simulink model "e02_MtrCtrl_Pst"  (R2024a)
settings: Solver=FixedStepDiscrete  StartTime=0.0  StopTime=1  FixedStep=mSim.dTime  MaxStep=Define.sModelSampleTime  RelTol=7.1420e-05
undefined symbols (not defined in the file): CnstCnst, E02ITDC, E02PST
libraries: simulink x6, Lib_LPF x3
settings Model: Creator=user  LastModifiedBy=admin
settings SolverCC: MaxConsecutiveZCs=10000  ZeroCrossAlgorithm=Adaptive  AlgebraicLoopSolver=TrustRegion
settings DataIOCC: SaveOutput=off  DSMLogging=off  InspectSignalLogs=on  SaveTime=off  SignalLoggingName=logsout_Validator
settings OptimizationCC: BlockReduction=off  DefaultParameterBehavior=Inlined  UseDivisionForNetSlopeComputation=UseDivisionForReciprocalsOfIntegersOnly  GainParamInheritBuiltInType=on  UseFloatMulNetSlope=on  DefaultUnderspecifiedDataType=single  InlineInvariantSignals=on  BitwiseOrLogicalOp=Logical operator  PassReuseOutputArgsAs=Individual arguments  EfficientFloat2IntCast=on  LifeSpan=Inf  OptimizeBlockOrder=speed  DifferentSizesBufferReuse=on  EfficientTunableParamExpr=on
settings DebuggingCC: SignalInfNanChecking=error  SignalRangeChecking=error  ReadBeforeWriteMsg=EnableAllAsError  WriteAfterWriteMsg=EnableAllAsError  WriteAfterReadMsg=EnableAllAsError  AlgebraicLoopMsg=error  ArtificialAlgebraicLoopMsg=error  SaveWithDisabledLinksMsg=error  SaveWithParameterizedLinksMsg=error  BlockPriorityViolationMsg=error  SolverPrmCheckMsg=error  InheritedTsInSrcMsg=error  SingleTaskRateTransMsg=error  TasksWithSamePriorityMsg=error  SigSpecEnsureSampleTimeMsg=error  CheckMatrixSingularityMsg=error  IntegerOverflowMsg=error  ParameterUnderflowMsg=error  ParameterPrecisionLossMsg=error  ParameterTunabilityLossMsg=error  UnderSpecifiedDataTypeMsg=error  UnnecessaryDatatypeConvMsg=warning  VectorMatrixConversionMsg=error  SignalLabelMismatchMsg=error  UnconnectedInputMsg=error  UnconnectedOutputMsg=error  UnconnectedLineMsg=error  SFcnCompatibilityMsg=error  UniqueDataStoreMsg=error  BusObjectLabelMismatch=error  RootOutportRequireBusObject=error  AssertControl=DisableAll  ModelReferenceIOMismatchMessage=error  UnknownTsInhSupMsg=error  ModelReferenceDataLoggingMessage=error  ModelReferenceSymbolNameMessage=none  StateNameClashWarn=warning  StrictBusMsg=ErrorOnBusTreatedAsVector  NonBusSignalsTreatedAsBus=error  SFInvalidInputDataAccessInChartInitDiag=error  SFTransitionOutsideNaturalParentDiag=error  SFUnreachableExecutionPathDiag=error  SFUndirectedBroadcastEventsDiag=error  SFTransitionActionBeforeConditionDiag=error  SFTemporalDelaySmallerThanSampleTimeDiag=error  SFSelfTransitionDiag=error  SFExecutionAtInitializationDiag=error  IntegerSaturationMsg=error  UnitsInconsistencyMsg=none  VariantConditionMismatch=error
settings HardwareCC: ProdBitPerChar=16  ProdBitPerInt=16  ProdBitPerPointer=32  ProdBitPerSizeT=32  ProdBitPerPtrDiffT=32  ProdLargestAtomicInteger=Integer  ProdLargestAtomicFloat=None  ProdWordSize=16  ProdLongLongMode=on  ProdHWDeviceType=Texas Instruments->C2000
settings ModelReferenceCC: EnableRefExpFcnMdlSchedulingChecks=on  ModelReferenceNumInstancesAllowed=Single
settings SFSimCC: SimUseLocalCustomCode=off  CompileTimeRecursionLimit=0  EnableRuntimeRecursion=off  MATLABDynamicMemAlloc=off  CustomCodeUndefinedFunction=UseInterfaceOnly
settings RTWCC: Description=Embedded Coder  SystemTargetFile=ert.tlc  GenCodeOnly=on  TemplateMakefile=ert_default_tmf  GenerateReport=on  RTWUseLocalCustomCode=off  BuildConfiguration=Faster Runs  IncludeHyperlinkInReport=on  LaunchReport=on  GenerateTraceInfo=on  GenerateTraceReport=on  GenerateTraceReportSl=on  GenerateTraceReportSf=on  GenerateWebview=on  GenerateCodeMetricsReport=on  GenerateCodeReplacementReport=on  GPUComputeCapability=3.5  DLArmComputeVersion=19.05
settings CodeAppCC: ForceParamTrailComments=on  IgnoreCustomStorageClasses=off  MATLABFcnDesc=on  MangleLength=4  CustomSymbolStrGlobalVar=GvE02$N$M  CustomSymbolStrType=StrE02$N$M  CustomSymbolStrFcn=$N$M$F  CustomSymbolStrMacro=$N$M  DefineNamingRule=UpperCase  ParamNamingRule=UpperCase  SimulinkBlockComments=off  MATLABSourceComments=on  EnableCustomComments=on  ReqsInCode=on
settings ERTTargetCC: TargetLangStandard=C99 (ISO)  UtilityFuncGeneration=Shared location  MultiwordLength=2048  IncludeMdlTerminateFcn=off  CombineSignalStateStructs=on  SuppressErrorStatus=on  SupportAbsoluteTime=off  SupportNonFinite=off  ParenthesesLevel=Maximum  CastingMode=Standards  GenerateSharedConstants=off  InlinedParameterPlacement=NonHierarchical  ERTSrcFileBannerTemplate=t_code_template.cgt  ERTHdrFileBannerTemplate=t_code_template.cgt  ERTDataSrcFileTemplate=t_code_template.cgt  ERTDataHdrFileTemplate=t_code_template.cgt  ERTCustomFileTemplate=example_file_process.tlc  ERTFilePackagingFormat=CompactWithDataFile  PreserveExpressionOrder=on  SuppressUnreachableDefaultCases=off  EnableSignedLeftShifts=off  EnableSignedRightShifts=off  IndentStyle=Allman  IndentSize=4
settings ConfigComp: CovSaveName=coveragedata  CovMetricSettings=we  CovEnableCumulative=off  CovSaveCumulativeToWorkspaceVar=on  CovSaveSingleToWorkspaceVar=on  CovOutputDir=sldv_output/$ModelName$\sldv_covoutput  PSVerificationMode=BugFinder  PSModelRefIgnoreList=[]  PSEnableModelRefIgnoreList=off  PSModelRefMinMaxVerif=CheckAndConstrain  PSAutoStubLUT=on  DVModelCoverageObjectives=MCDC  DVTestSuiteOptimization=CombinedObjectives (Nonlinear Extended)  DVRebuildModelRepresentation=Always
settings SimscapeCC: SimscapeNormalizeSystem=off

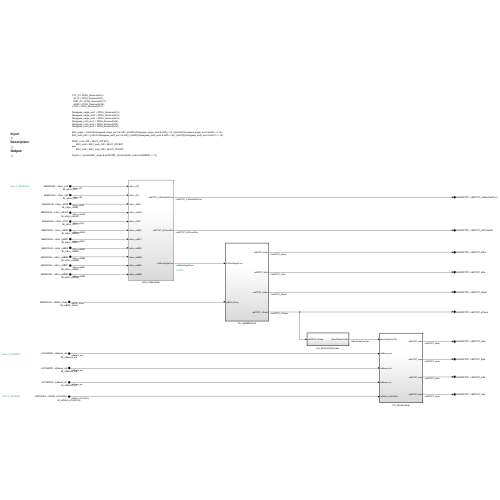
[thumbnail: Simulink's stored preview of the top-level diagram]
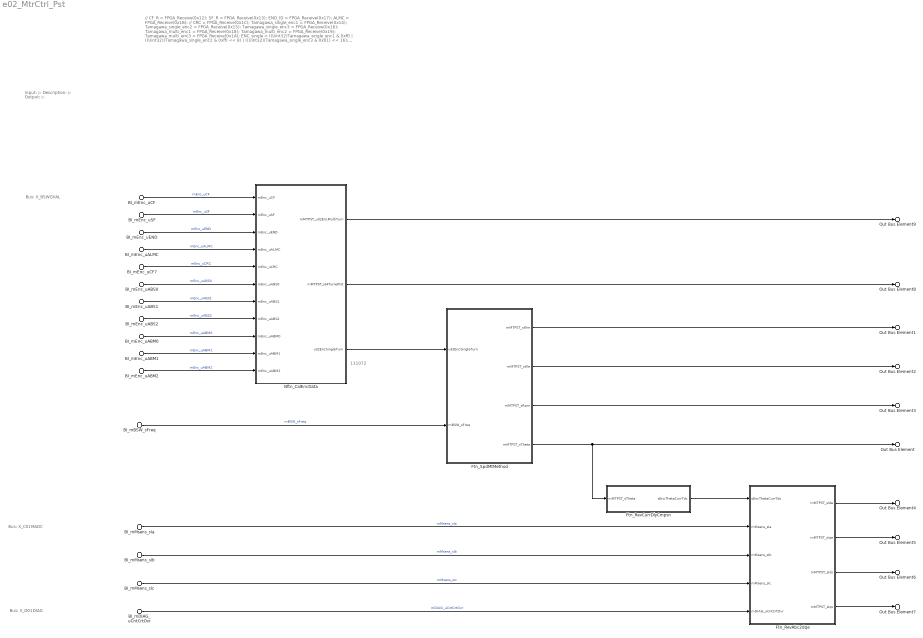
== system e02_MtrCtrl_Pst ==
  note: Bus: X_C01MADC
  note: Bus: X_BSWGVAL
  note: 131072
  note: Input:
      | ▷
      | Description:
      | ▷
      | Output:
      | ▷
  note: // CF_R = FPGA_Receive(0x12);
      |    SF_R = FPGA_Receive(0x13);
      |    END_ID = FPGA_Receive(0x17);
      |    ALMC = FPGA_Receive(0x1B);
      | // CRC = FPGA_Receive(0x1C);
      |
      | Tamagawa_single_enc1 = FPGA_Receive(0x14);
      | Tamagawa_single_enc2 = FPGA_Receive(0x15);
      | Tamagawa_single_enc3 = FPGA_Receive(0x16);
      | Tamagawa_multi_enc1 = FPGA_Receive(0x18);
      | Tamagawa_multi_enc2 = FPGA_Receive(0x19);
      | Tamagawa_multi_enc3 = FPGA_Receive(0x1A);
      |
      | ENC_single = ((Uint32)Tamagawa_single_enc1 & 0xff) | ((Uint32)(Tamagawa_single_enc2 & 0xff) << 8) | ((Uint32)(Tamagawa_single_enc3 & 0x01) << 16);
      | ENC_multi_ORI = ((Uint32)Tamagawa_multi_enc1 & 0xff) | ((Uint32)(Tamagawa_multi_enc2 & 0xff) << 8) | ((Uint32)(Tamagawa_multi_enc3 & 0x01) << 16);
      |
      | if(ENC_multi_ORI > MULTI_OFFSET)
      | 	ENC_multi = ENC_multi_ORI - MULTI_OFFSET;
      | else
      | 	ENC_multi = ENC_multi_ORI + MULTI_OFFSET;
      |
      | Position = ((Uint64)ENC_single & 0x0001ffff) | ((Uint64)(ENC_multi & 0x0000ffff) << 17);
  note: Bus: X_D01DIAG
  BI_mBSW_sFreq : Inport  Description=■ 설명: 제어 주파수  PortName=bBSWGVAL  Element=mBSW_sFreq
  BI_mEnc_uCF : Inport  Description=■ 설명: Control Field  PortName=bBSWGVAL  Element=mEnc_uCF
  BI_mEnc_uSF : Inport  Description=■ 설명: Status Field  PortName=bBSWGVAL  Element=mEnc_uSF
  BI_mEnc_uEND : Inport  Description=■ 설명: 엔코더 ID (= 23H 고정)  PortName=bBSWGVAL  Element=mEnc_uEND
  BI_mEnc_uALMC : Inport  Description=■ 설명: 인코더 오류  PortName=bBSWGVAL  Element=mEnc_uALMC
  BI_mEnc_uCF7 : Inport  Description=■ 설명: 생성 식 G (X) = X^8 + 1 (X = rc0 ~ rc7)  PortName=bBSWGVAL  Element=mEnc_uCRC
  BI_mEnc_uABS0 : Inport  Description=■ 설명: Data Field 0  PortName=bBSWGVAL  Element=mEnc_uABS0
  BI_mEnc_uABS1 : Inport  Description=■ 설명: Data Field 1  PortName=bBSWGVAL  Element=mEnc_uABS1
  BI_mEnc_uABS2 : Inport  Description=■ 설명: Data Field 2  PortName=bBSWGVAL  Element=mEnc_uABS2
  BI_mEnc_uABM0 : Inport  Description=■ 설명: Data Field 4  PortName=bBSWGVAL  Element=mEnc_uABM0
  BI_mEnc_uABM1 : Inport  Description=■ 설명: Data Field 5  PortName=bBSWGVAL  Element=mEnc_uABM1
  BI_mEnc_uABM2 : Inport  Description=■ 설명: Data Field 6  PortName=bBSWGVAL  Element=mEnc_uABM2
  BI_mMsens_sIa : Inport  Description=■ 설명: A상 전류  Port=2  PortName=bC01MADC  Element=mMsens_sIa
  BI_mMsens_sIb : Inport  Description=■ 설명: B상 전류  Port=2  PortName=bC01MADC  Element=mMsens_sIb
  BI_mMsens_sIc : Inport  Description=■ 설명: C상 전류  Port=2  PortName=bC01MADC  Element=mMsens_sIc
  BI_mDIAG_uCntCrtOvr : Inport  Description=■ 설명: 과전류 검출 카운터  Port=3  PortName=bD01DIAG  Element=mDIAG_uCntCrtOvr
  Ftn_RevAbc2dqe : Subsystem  Description=DQ Transformation  Priority=1  TreatAsAtomicUnit=on
      settings: RTWSystemCode=Nonreusable function  RTWFcnNameOpts=Use subsystem name
  Ftn_RevCurrDlyCmpsn : Subsystem  TreatAsAtomicUnit=on
      settings: RTWSystemCode=Nonreusable function  RTWFcnNameOpts=Use subsystem name
  Ftn_SpdMtMethod : Subsystem  TreatAsAtomicUnit=on
      settings: RTWSystemCode=Nonreusable function  RTWFcnNameOpts=Use subsystem name
  Nftn_CalEncData : Subsystem
      settings: RTWSystemCode=Nonreusable function  RTWFcnNameOpts=Use subsystem name
  Out Bus Element1 : Outport  Description=■ 설명: 기계 각속도 (Wm = 12000 * 2pi/60)  PortName=bE02MTPST  Element=mMTPST_sWm
  Out Bus Element2 : Outport  Description=■ 설명: 기계 각속도 (We = 10000 * 2pi/60 * Poles)  PortName=bE02MTPST  Element=mMTPST_sWe
  Out Bus Element3 : Outport  Description=■ 설명: Motor Speed  PortName=bE02MTPST  Element=mMTPST_sRpm
  Out Bus Element : Outport  Description=■ 설명: Rotor Position  PortName=bE02MTPST  Element=mMTPST_sTheta
  Out Bus Element9 : Outport  Description=■ 설명: 엔코더 멀티턴 수신 값  PortName=bE02MTPST  Element=mMTPST_u32EncMultiTurn
  Out Bus Element8 : Outport  Description=■ 설명: Turret Position  PortName=bE02MTPST  Element=mMTPST_i64TurretPst
  Out Bus Element4 : Outport  Description=■ 설명: 기계 각속도 (Wm = 12000 * 2pi/60)  PortName=bE02MTPST  Element=mMTPST_sIde
  Out Bus Element5 : Outport  Description=■ 설명: 기계 각속도 (We = 10000 * 2pi/60 * Poles)  PortName=bE02MTPST  Element=mMTPST_sIqe
  Out Bus Element6 : Outport  Description=■ 설명: Motor Speed  PortName=bE02MTPST  Element=mMTPST_sIds
  Out Bus Element7 : Outport  Description=■ 설명: Rotor Position  PortName=bE02MTPST  Element=mMTPST_sIqs
  wires:
  Ftn_SpdMtMethod/3(mMTPST_sRpm) -> Out Bus Element3/1
  Ftn_SpdMtMethod/2(mMTPST_sWe) -> Out Bus Element2/1
  BI_mBSW_sFreq/1 -> Ftn_SpdMtMethod/2(mBSW_sFreq)  "mBSW_sFreq"
  Ftn_SpdMtMethod/4(mMTPST_sTheta) -> Out Bus Element/1, Ftn_RevCurrDlyCmpsn/1(mMTPST_sTheta)
  Ftn_SpdMtMethod/1(mMTPST_sWm) -> Out Bus Element1/1
  Ftn_RevCurrDlyCmpsn/1(sEncThetaCurrTdc) -> Ftn_RevAbc2dqe/1(sEncThetaCurrTdc)
  BI_mMsens_sIa/1 -> Ftn_RevAbc2dqe/2(mMsens_sIa)  "mMsens_sIa"
  BI_mMsens_sIb/1 -> Ftn_RevAbc2dqe/3(mMsens_sIb)  "mMsens_sIb"
  BI_mMsens_sIc/1 -> Ftn_RevAbc2dqe/4(mMsens_sIc)  "mMsens_sIc"
  BI_mDIAG_uCntCrtOvr/1 -> Ftn_RevAbc2dqe/5(mDIAG_uCntCrtOvr)  "mDIAG_uCntCrtOvr"
  Ftn_RevAbc2dqe/1(mMTPST_sIde) -> Out Bus Element4/1
  Ftn_RevAbc2dqe/2(mMTPST_sIqe) -> Out Bus Element5/1
  Ftn_RevAbc2dqe/3(mMTPST_sIds) -> Out Bus Element6/1
  Ftn_RevAbc2dqe/4(mMTPST_sIqs) -> Out Bus Element7/1
  BI_mEnc_uCF/1 -> Nftn_CalEncData/1(mEnc_uCF)  "mEnc_uCF"
  BI_mEnc_uSF/1 -> Nftn_CalEncData/2(mEnc_uSF)  "mEnc_uSF"
  BI_mEnc_uEND/1 -> Nftn_CalEncData/3(mEnc_uEND)  "mEnc_uEND"
  BI_mEnc_uALMC/1 -> Nftn_CalEncData/4(mEnc_uALMC)  "mEnc_uALMC"
  BI_mEnc_uCF7/1 -> Nftn_CalEncData/5(mEnc_uCRC)  "mEnc_uCRC"
  BI_mEnc_uABS0/1 -> Nftn_CalEncData/6(mEnc_uABS0)  "mEnc_uABS0"
  BI_mEnc_uABS1/1 -> Nftn_CalEncData/7(mEnc_uABS1)  "mEnc_uABS1"
  BI_mEnc_uABS2/1 -> Nftn_CalEncData/8(mEnc_uABS2)  "mEnc_uABS2"
  BI_mEnc_uABM0/1 -> Nftn_CalEncData/9(mEnc_uABM0)  "mEnc_uABM0"
  BI_mEnc_uABM1/1 -> Nftn_CalEncData/10(mEnc_uABM1)  "mEnc_uABM1"
  BI_mEnc_uABM2/1 -> Nftn_CalEncData/11(mEnc_uABM2)  "mEnc_uABM2"
  Nftn_CalEncData/2(mMTPST_i64TurretPst) -> Out Bus Element8/1
  Nftn_CalEncData/3(u32EncSingleTurn) -> Ftn_SpdMtMethod/1(u32EncSingleTurn)
  Nftn_CalEncData/1(mMTPST_u32EncMultiTurn) -> Out Bus Element9/1

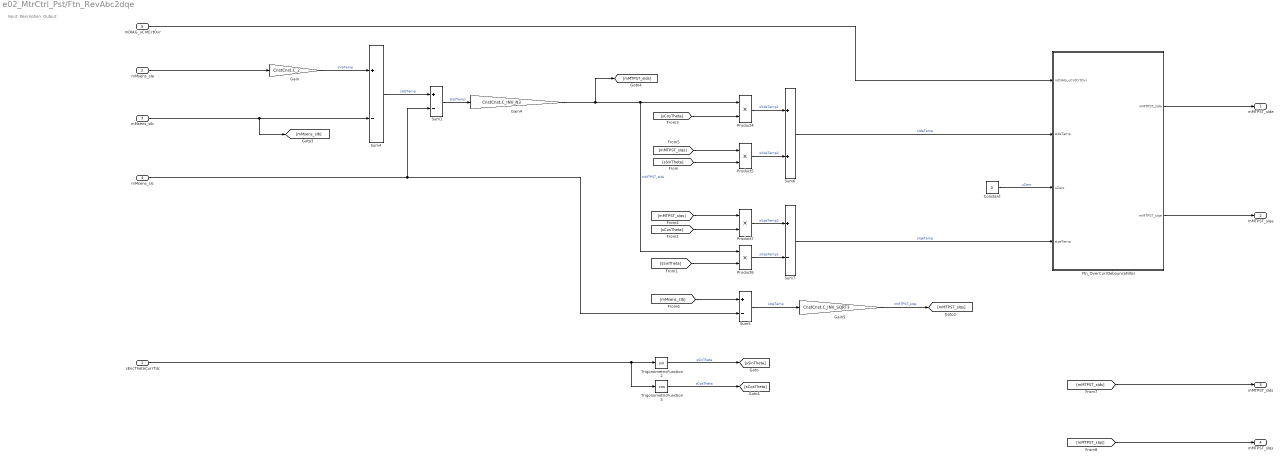
== system e02_MtrCtrl_Pst/Ftn_RevAbc2dqe ==
  note: Input:
      | Description:
      | Output:
  sEncThetaCurrTdc : Inport  Description=■ 설명: 회전자 위치 (전류 시지연 보상 후)  OutMin=0  OutMax=6.2832
      settings: AttributesFormatString=%<Description>
  mMsens_sIa : Inport  Description=■ 설명: 모터 A상 전류  Port=2  OutMin=-162.6  OutMax=162.6
      settings: AttributesFormatString=%<Description>
  mMsens_sIb : Inport  Description=■ 설명: 모터 B상 전류  Port=3  OutMin=-162.6  OutMax=162.6
      settings: AttributesFormatString=%<Description>
  mMsens_sIc : Inport  Description=■ 설명: 모터 C상 전류  Port=4  OutMin=-325.2  OutMax=325.2
      settings: AttributesFormatString=%<Description>
  mDIAG_uCntCrtOvr : Inport  Description=■ 설명: 과전류 발생 카운트 신호  Port=5  OutMin=0  OutMax=2
      settings: AttributesFormatString=%<Description>
  Constant : Constant  Value=0  OutDataTypeStr=uint16
  Ftn_OverCurrDebounceFilter : Stateflow chart
  Gain : Gain  Gain=CnstCnst.C_2
  Gain4 : Gain  Gain=CnstCnst.C_INV_N3
  Gain5 : Gain  Gain=CnstCnst.C_INV_SQRT3
  Product{4..7} (4 alike) : Product  RndMeth=Zero
  Sum{1,4..5,7} (4 alike) : Sum  Inputs=+-
  Sum6 : Sum
  TrigonometricFunction2 : Trigonometry
  TrigonometricFunction3 : Trigonometry  Operator=cos
  mMTPST_sIde : Outport  Description=■ 설명: d축 전류 ( 회전 좌표계 )  OutMin=-398.3  OutMax=398.3
      settings: AttributesFormatString=%<Description>
  mMTPST_sIqe : Outport  Description=■ 설명: q축 전류 ( 회전 좌표계 )  Port=2  OutMin=-398.3  OutMax=398.3
      settings: AttributesFormatString=%<Description>
  mMTPST_sIds : Outport  Description=■ 설명: d축 전류 ( 정지 좌표계 )  Port=3  OutMin=-271  OutMax=271
      settings: AttributesFormatString=%<Description>
  mMTPST_sIqs : Outport  Description=■ 설명: q축 전류 ( 정지 좌표계 )  Port=4  OutMin=-271  OutMax=271
      settings: AttributesFormatString=%<Description>
  wires:
  mDIAG_uCntCrtOvr/1 -> Ftn_OverCurrDebounceFilter/1(mDIAG_uCntCrtOvr)
  Ftn_OverCurrDebounceFilter/2(mMTPST_sIqe) -> mMTPST_sIqe/1
  Ftn_OverCurrDebounceFilter/1(mMTPST_sIde) -> mMTPST_sIde/1
  [mMTPST_sIqs] -> Product7/1
  Gain5/1 -> [mMTPST_sIqs]  "mMTPST_sIqs"
  sEncThetaCurrTdc/1 -> TrigonometricFunction3/1, TrigonometricFunction2/1
  [sCosTheta] -> Product7/2
  Gain4/1 -> [mMTPST_sIds], Product6/1, Product4/1  "mMTPST_sIds"
  [sSinTheta] -> Product6/2
  [mMsens_sIb] -> Sum5/1
  mMsens_sIb/1 -> [mMsens_sIb], Sum4/2
  Sum5/1 -> Gain5/1  "sIqsTemp"
  mMsens_sIa/1 -> Gain/1
  Sum1/1 -> Gain4/1  "sIdsTemp"
  mMsens_sIc/1 -> Sum1/2, Sum5/2
  Gain/1 -> Sum4/1  "sVaTemp"
  TrigonometricFunction2/1 -> [sSinTheta]  "sSinTheta"
  Product7/1 -> Sum7/1  "sVqeTemp2"
  Product4/1 -> Sum6/1  "sVdeTemp1"
  [mMTPST_sIqs] -> Product5/1
  Product5/1 -> Sum6/2  "sVdeTemp2"
  Product6/1 -> Sum7/2  "sVqeTemp1"
  [sCosTheta] -> Product4/2
  [sSinTheta] -> Product5/2
  Sum7/1 -> Ftn_OverCurrDebounceFilter/4(sIqeTemp)  "sIqeTemp"
  TrigonometricFunction3/1 -> [sCosTheta]  "sCosTheta"
  Sum6/1 -> Ftn_OverCurrDebounceFilter/2(sIdeTemp)  "sIdeTemp"
  [mMTPST_sIds] -> mMTPST_sIds/1
  [mMTPST_sIqs] -> mMTPST_sIqs/1
  Constant/1 -> Ftn_OverCurrDebounceFilter/3(uZero)  "uZero"
  Sum4/1 -> Sum1/1  "sIdsTemp"

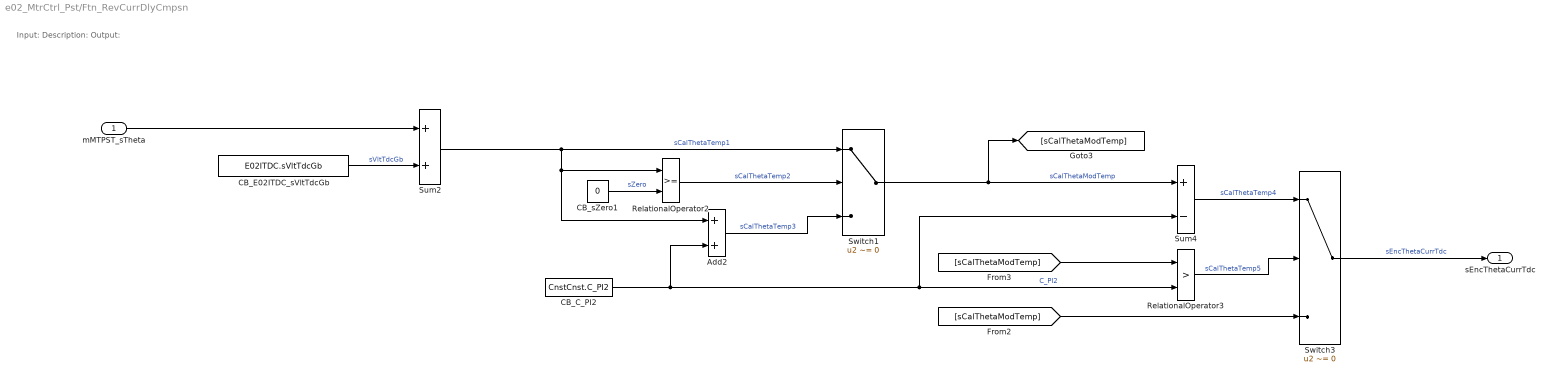
== system e02_MtrCtrl_Pst/Ftn_RevCurrDlyCmpsn ==
  note: Input:
      | Description:
      | Output:
  mMTPST_sTheta : Inport  Description=■ 설명: 회전자 위치  OutMin=0  OutMax=6.2832
      settings: AttributesFormatString=%<Description>
  Add2 : Sum
  CB_C_PI2 : Constant  Value=CnstCnst.C_PI2
  CB_E02ITDC_sVltTdcGb : Constant  Value=E02ITDC.sVltTdcGb  OutDataTypeStr=single
  CB_sZero1 : Constant  Value=0  OutDataTypeStr=single
  RelationalOperator2 : RelationalOperator  InputSameDT=off
  RelationalOperator3 : RelationalOperator  Operator=>  InputSameDT=off
  Sum2 : Sum
  Sum4 : Sum  Inputs=+-
  Switch1 : Switch  Criteria=u2 ~= 0  SaturateOnIntegerOverflow=off  InputSameDT=off
  Switch3 : Switch  Criteria=u2 ~= 0  SaturateOnIntegerOverflow=off  InputSameDT=off
  sEncThetaCurrTdc : Outport  Description=■ 설명: 회전자 위치 (전류 시지연 보상 후)  OutMin=0  OutMax=6.2832
      settings: AttributesFormatString=%<Description>
  wires:
  mMTPST_sTheta/1 -> Sum2/1
  Switch3/1 -> sEncThetaCurrTdc/1  "sEncThetaCurrTdc"
  CB_E02ITDC_sVltTdcGb/1 -> Sum2/2  "sVltTdcGb"
  Sum4/1 -> Switch3/1  "sCalThetaTemp4"
  CB_C_PI2/1 -> Add2/2, RelationalOperator3/2, Sum4/2  "C_PI2"
  RelationalOperator2/1 -> Switch1/2  "sCalThetaTemp2"
  Switch1/1 -> Sum4/1, [sCalThetaModTemp]  "sCalThetaModTemp"
  CB_sZero1/1 -> RelationalOperator2/2  "sZero"
  RelationalOperator3/1 -> Switch3/2  "sCalThetaTemp5"
  [sCalThetaModTemp] -> RelationalOperator3/1
  [sCalThetaModTemp] -> Switch3/3
  Add2/1 -> Switch1/3  "sCalThetaTemp3"
  Sum2/1 -> Add2/1, RelationalOperator2/1, Switch1/1  "sCalThetaTemp1"

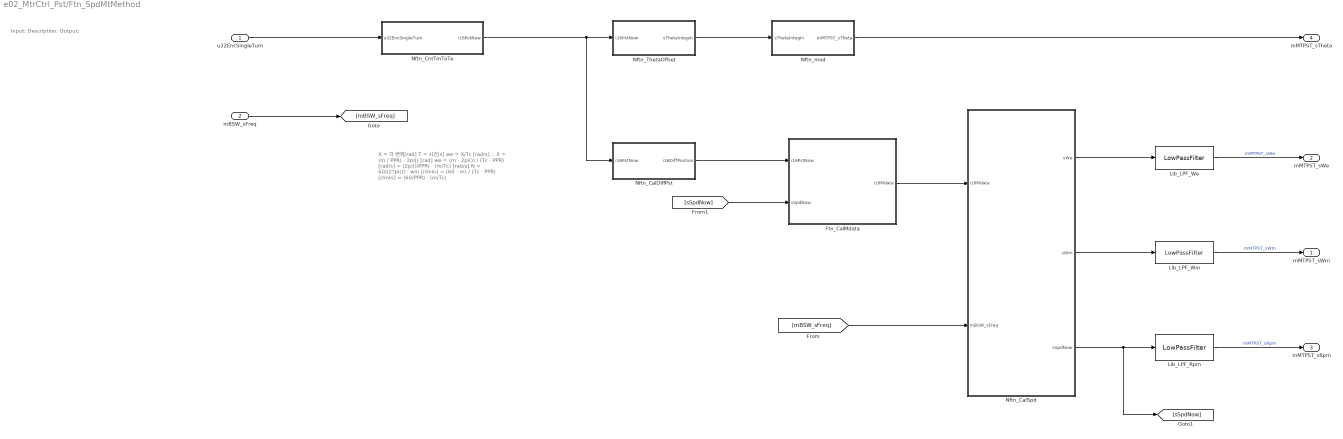
== system e02_MtrCtrl_Pst/Ftn_SpdMtMethod ==
  note: X = 각 변위[rad]
      | T = 시간[s]
      | we = X/Tc [rad/s]
      | ∴ X = (m / PPR) · 2pi() [rad]
      | we = (m · 2pi()) / (Tc · PPR) [rad/s]
      | = (2pi()/PPR) · (m/Tc) [rad/s]
      | N = 60/(2*pi()) · wm [r/min]
      | = (60 · m) / (Tc · PPR) [r/min]
      | = (60/PPR) · (m/Tc)
  note: Input:
      | Description:
      | Output:
  u32EncSingleTurn : Inport  Description=■ 설명: Resolver Count  OutMin=0  OutMax=131072
      settings: AttributesFormatString=%<Description>
  mBSW_sFreq : Inport  Description=■ 설명: Time base Frequency  Port=2  OutMin=0  OutMax=16000
      settings: AttributesFormatString=%<Description>
  Ftn_CalMdata : Subsystem  TreatAsAtomicUnit=on
      settings: RTWSystemCode=Nonreusable function  RTWFcnNameOpts=Use subsystem name
  Lib_LPF_Rpm : Lib_LPF/LowPassFilter  La=E02SWF.sEstSpdLa  Lb=E02SWF.sEstSpdLb  Init_Value=0
  Lib_LPF_We : Lib_LPF/LowPassFilter  La=E02SWF.sEstWeLa  Lb=E02SWF.sEstWeLb  Init_Value=0
  Lib_LPF_Wm : Lib_LPF/LowPassFilter  La=E02SWF.sEstWmLa  Lb=E02SWF.sEstWmLb  Init_Value=0
  Nftn_CalDiffPst : Subsystem
  Nftn_CalSpd : Subsystem
  Nftn_CntTmToTe : Subsystem
  Nftn_ThetaOffset : Subsystem
  Nftn_mod : Subsystem
  mMTPST_sWm : Outport  Description=■ 설명: 기계 각속도
      settings: AttributesFormatString=%<Description>
  mMTPST_sWe : Outport  Description=■ 설명: 전기 각속도  Port=2  OutMin=0  OutMax=5026.55
      settings: AttributesFormatString=%<Description>
  mMTPST_sRpm : Outport  Description=■ 설명: 속도  Port=3  OutMin=0  OutMax=12000
      settings: AttributesFormatString=%<Description>
  mMTPST_sTheta : Outport  Description=■ 설명: 회전자 위치  Port=4  OutMin=0  OutMax=6.2832
      settings: AttributesFormatString=%<Description>
  wires:
  Nftn_mod/1(mMTPST_sTheta) -> mMTPST_sTheta/1
  Nftn_CntTmToTe/1(i16PstNow) -> Nftn_CalDiffPst/1(i16PstNow), Nftn_ThetaOffset/1(i16PstNow)
  Nftn_CalDiffPst/1(i16DiffPostion) -> Ftn_CalMdata/1(i16PstNow)
  u32EncSingleTurn/1 -> Nftn_CntTmToTe/1(u32EncSingleTurn)
  Nftn_ThetaOffset/1(sThetaIntegIn) -> Nftn_mod/1(sThetaIntegIn)
  Nftn_CalSpd/3(sSpdNow) -> [sSpdNow], Lib_LPF_Rpm/1
  Ftn_CalMdata/1(i16Mdata) -> Nftn_CalSpd/1(i16Mdata)
  Nftn_CalSpd/1(sWe) -> Lib_LPF_We/1
  mBSW_sFreq/1 -> [mBSW_sFreq]
  [mBSW_sFreq] -> Nftn_CalSpd/2(mBSW_sFreq)
  [sSpdNow] -> Ftn_CalMdata/2(sSpdNow)
  Nftn_CalSpd/2(sWm) -> Lib_LPF_Wm/1
  Lib_LPF_We/1 -> mMTPST_sWe/1  "mMTPST_sWe"
  Lib_LPF_Wm/1 -> mMTPST_sWm/1  "mMTPST_sWm"
  Lib_LPF_Rpm/1 -> mMTPST_sRpm/1  "mMTPST_sRpm"

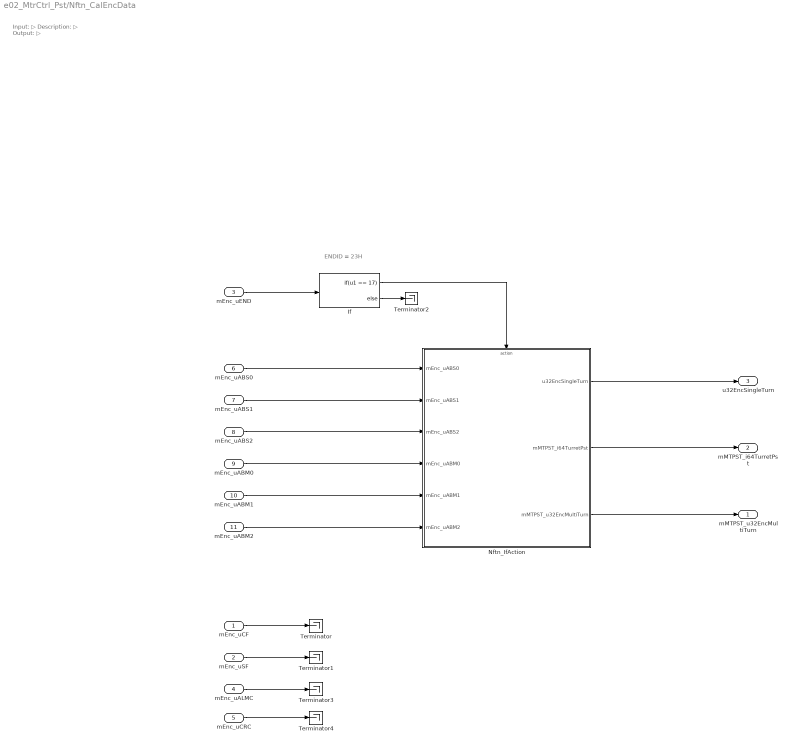
== system e02_MtrCtrl_Pst/Nftn_CalEncData ==
  note: ENDID = 23H
  note: Input:
      | ▷
      | Description:
      | ▷
      | Output:
      | ▷
  mEnc_uCF : Inport
  mEnc_uSF : Inport  Port=2
  mEnc_uEND : Inport  Port=3
  mEnc_uALMC : Inport  Port=4
  mEnc_uCRC : Inport  Port=5
  mEnc_uABS0 : Inport  Port=6
  mEnc_uABS1 : Inport  Port=7
  mEnc_uABS2 : Inport  Port=8
  mEnc_uABM0 : Inport  Port=9
  mEnc_uABM1 : Inport  Port=10
  mEnc_uABM2 : Inport  Port=11
  If : If  IfExpression=u1 == 17
  Nftn_IfAction : Subsystem
  Terminator{,1..4} (5 alike) : Terminator
  mMTPST_u32EncMultiTurn : Outport
  mMTPST_i64TurretPst : Outport  Port=2
  u32EncSingleTurn : Outport  Port=3  OutMin=0  OutMax=131072
  wires:
  mEnc_uCF/1 -> Terminator/1
  mEnc_uSF/1 -> Terminator1/1
  mEnc_uALMC/1 -> Terminator3/1
  mEnc_uEND/1 -> If/1
  mEnc_uCRC/1 -> Terminator4/1
  mEnc_uABS0/1 -> Nftn_IfAction/1(mEnc_uABS0)
  mEnc_uABS1/1 -> Nftn_IfAction/2(mEnc_uABS1)
  mEnc_uABS2/1 -> Nftn_IfAction/3(mEnc_uABS2)
  mEnc_uABM0/1 -> Nftn_IfAction/4(mEnc_uABM0)
  mEnc_uABM1/1 -> Nftn_IfAction/5(mEnc_uABM1)
  mEnc_uABM2/1 -> Nftn_IfAction/6(mEnc_uABM2)
  Nftn_IfAction/1(u32EncSingleTurn) -> u32EncSingleTurn/1
  Nftn_IfAction/2(mMTPST_i64TurretPst) -> mMTPST_i64TurretPst/1
  If/2 -> Terminator2/1
  If/1 -> Nftn_IfAction/Action
  Nftn_IfAction/3(mMTPST_u32EncMultiTurn) -> mMTPST_u32EncMultiTurn/1

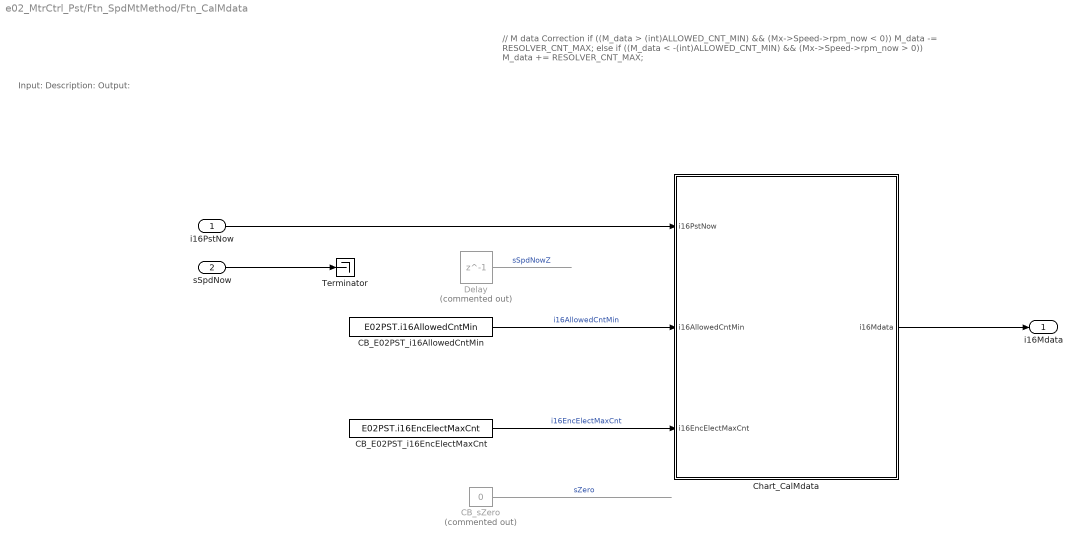
== system e02_MtrCtrl_Pst/Ftn_SpdMtMethod/Ftn_CalMdata ==
  note: // M data Correction
      | if ((M_data > (int)ALLOWED_CNT_MIN) && (Mx->Speed->rpm_now < 0))
      | M_data -= RESOLVER_CNT_MAX;
      | else if ((M_data < -(int)ALLOWED_CNT_MIN) && (Mx->Speed->rpm_now > 0))
      | M_data += RESOLVER_CNT_MAX;
  note: Input:
      | Description:
      | Output:
  i16PstNow : Inport  Description=■ 설명: 위치 센서 변위 값  OutMin=-4095  OutMax=4095
      settings: AttributesFormatString=%<Description>
  sSpdNow : Inport  Port=2
  CB_E02PST_i16AllowedCntMin : Constant  Value=E02PST.i16AllowedCntMin
  CB_E02PST_i16EncElectMaxCnt : Constant  Value=E02PST.i16EncElectMaxCnt
  CB_sZero : Constant  Commented=on  Value=0  OutDataTypeStr=single
  Chart_CalMdata : Stateflow chart  TreatAsAtomicUnit=on
  Delay : Delay  Commented=on  DelayLength=1
  Terminator : Terminator
  i16Mdata : Outport  Description=■ 설명: 속도 추종 값에 해당하는 센서 값  OutMin=0  OutMax=4095
      settings: AttributesFormatString=%<Description>
  wires:
  Chart_CalMdata/1(i16Mdata) -> i16Mdata/1
  sSpdNow/1 -> Terminator/1
  i16PstNow/1 -> Chart_CalMdata/1(i16PstNow)
  CB_sZero/1 -> ?  "sZero"
  CB_E02PST_i16AllowedCntMin/1 -> Chart_CalMdata/2(i16AllowedCntMin)  "i16AllowedCntMin"
  CB_E02PST_i16EncElectMaxCnt/1 -> Chart_CalMdata/3(i16EncElectMaxCnt)  "i16EncElectMaxCnt"
  Delay/1 -> ?  "sSpdNowZ"

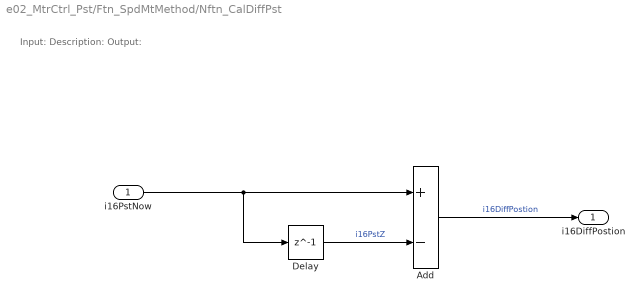
== system e02_MtrCtrl_Pst/Ftn_SpdMtMethod/Nftn_CalDiffPst ==
  note: Input:
      | Description:
      | Output:
  i16PstNow : Inport  Description=■ 설명: 위치센서 카운트 신호 ( NOW )  OutMin=0  OutMax=4095
      settings: AttributesFormatString=%<Description>
  Add : Sum  Inputs=+-
  Delay : Delay  DelayLength=1  StateName=i32PstZ
  i16DiffPostion : Outport  Description=■ 설명: 위치 센서 변위 값  OutMin=-4095  OutMax=4095
      settings: AttributesFormatString=%<Description>
  wires:
  i16PstNow/1 -> Add/1, Delay/1
  Delay/1 -> Add/2  "i16PstZ"
  Add/1 -> i16DiffPostion/1  "i16DiffPostion"

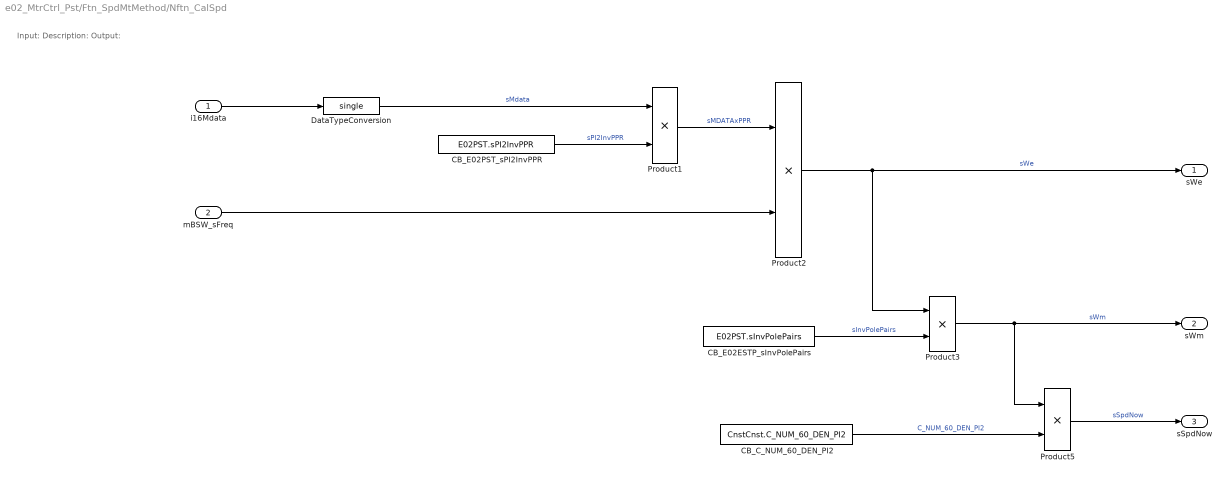
== system e02_MtrCtrl_Pst/Ftn_SpdMtMethod/Nftn_CalSpd ==
  note: Input:
      | Description:
      | Output:
  i16Mdata : Inport  Description=■ 설명: 속도 추종 값에 해당하는 센서 값  OutMin=0  OutMax=4095
      settings: AttributesFormatString=%<Description>
  mBSW_sFreq : Inport  Description=■ 설명: 스위칭 주파수  Port=2  OutMin=0  OutMax=14002
      settings: AttributesFormatString=%<Description>
  CB_C_NUM_60_DEN_PI2 : Constant  Value=CnstCnst.C_NUM_60_DEN_PI2
  CB_E02ESTP_sInvPolePairs : Constant  Value=E02PST.sInvPolePairs
  CB_E02PST_sPI2InvPPR : Constant  Value=E02PST.sPI2InvPPR
  DataTypeConversion : DataTypeConversion  OutDataTypeStr=single  SaturateOnIntegerOverflow=off  RndMeth=Floor
  Product{1..3,5} (4 alike) : Product
  sWe : Outport  Description=■ 설명: 전기 각속도  OutMin=0  OutMax=5026.55
      settings: AttributesFormatString=%<Description>
  sWm : Outport  Description=■ 설명: 기계 각속도  Port=2  OutMin=0  OutMax=1256.6371
      settings: AttributesFormatString=%<Description>
  sSpdNow : Outport  Description=■ 설명: 속도  Port=3  OutMin=0  OutMax=12000
      settings: AttributesFormatString=%<Description>
  wires:
  Product2/1 -> Product3/1, sWe/1  "sWe"
  i16Mdata/1 -> DataTypeConversion/1
  CB_C_NUM_60_DEN_PI2/1 -> Product5/2  "C_NUM_60_DEN_PI2"
  Product3/1 -> sWm/1, Product5/1  "sWm"
  CB_E02ESTP_sInvPolePairs/1 -> Product3/2  "sInvPolePairs"
  CB_E02PST_sPI2InvPPR/1 -> Product1/2  "sPI2InvPPR"
  Product1/1 -> Product2/1  "sMDATAxPPR"
  mBSW_sFreq/1 -> Product2/2
  Product5/1 -> sSpdNow/1  "sSpdNow"
  DataTypeConversion/1 -> Product1/1  "sMdata"

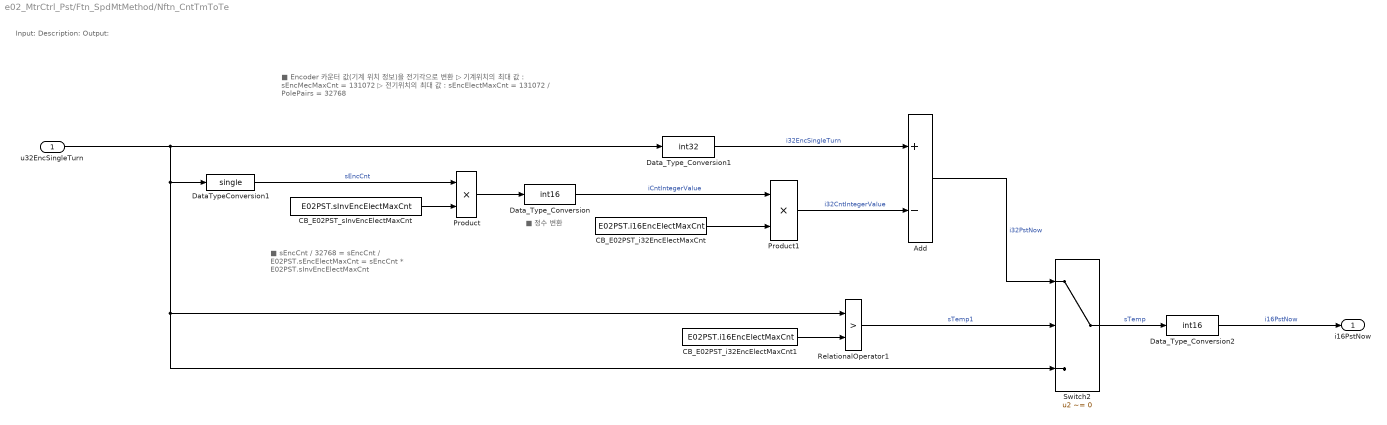
== system e02_MtrCtrl_Pst/Ftn_SpdMtMethod/Nftn_CntTmToTe ==
  note: ■ sEncCnt / 32768
      |
      | = sEncCnt / E02PST.sEncElectMaxCnt
      |
      | = sEncCnt * E02PST.sInvEncElectMaxCnt
  note: ■ Encoder 카운터 값(기계 위치 정보)을 전기각으로 변환
      | ▷ 기계위치의 최대 값 : sEncMecMaxCnt = 131072
      | ▷ 전기위치의 최대 값 : sEncElectMaxCnt = 131072 / PolePairs = 32768
  note: Input:
      | Description:
      | Output:
  note: ■ 정수 변환
  u32EncSingleTurn : Inport  Description=■ 설명: 위치센서 카운트 신호  OutMin=0  OutMax=4095
      settings: AttributesFormatString=%<Description>
  Add : Sum  Inputs=+-
  CB_E02PST_i32EncElectMaxCnt : Constant  Value=E02PST.i16EncElectMaxCnt
  CB_E02PST_i32EncElectMaxCnt1 : Constant  Value=E02PST.i16EncElectMaxCnt
  CB_E02PST_sInvEncElectMaxCnt : Constant  Value=E02PST.sInvEncElectMaxCnt
  DataTypeConversion1 : DataTypeConversion  OutDataTypeStr=single  SaturateOnIntegerOverflow=off  RndMeth=Floor
  Data_Type_Conversion : DataTypeConversion  OutDataTypeStr=int16  SaturateOnIntegerOverflow=off  RndMeth=Floor
  Data_Type_Conversion1 : DataTypeConversion  OutDataTypeStr=int32  SaturateOnIntegerOverflow=off  RndMeth=Floor
  Data_Type_Conversion2 : DataTypeConversion  OutDataTypeStr=int16  SaturateOnIntegerOverflow=off  RndMeth=Floor
  Product : Product
  Product1 : Product  OutDataTypeStr=int32
  RelationalOperator1 : RelationalOperator  Operator=>  InputSameDT=off
  Switch2 : Switch  Criteria=u2 ~= 0  SaturateOnIntegerOverflow=off  InputSameDT=off
  i16PstNow : Outport  Description=■ 설명: 위치센서 카운트 신호  OutMin=0  OutMax=4095
      settings: AttributesFormatString=%<Description>
  wires:
  Data_Type_Conversion/1 -> Product1/1  "iCntIntegerValue"
  Product/1 -> Data_Type_Conversion/1
  CB_E02PST_sInvEncElectMaxCnt/1 -> Product/2
  CB_E02PST_i32EncElectMaxCnt/1 -> Product1/2
  Add/1 -> Switch2/1  "i32PstNow"
  Switch2/1 -> Data_Type_Conversion2/1  "sTemp"
  RelationalOperator1/1 -> Switch2/2  "sTemp1"
  CB_E02PST_i32EncElectMaxCnt1/1 -> RelationalOperator1/2
  u32EncSingleTurn/1 -> RelationalOperator1/1, Switch2/3, DataTypeConversion1/1, Data_Type_Conversion1/1
  Data_Type_Conversion2/1 -> i16PstNow/1  "i16PstNow"
  DataTypeConversion1/1 -> Product/1  "sEncCnt"
  Product1/1 -> Add/2  "i32CntIntegerValue"
  Data_Type_Conversion1/1 -> Add/1  "i32EncSingleTurn"

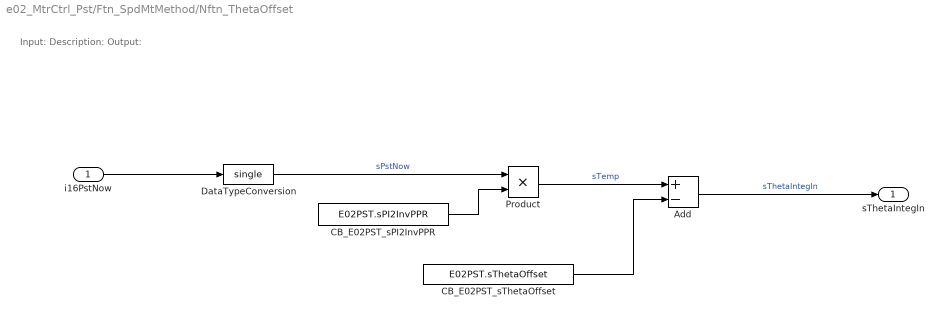
== system e02_MtrCtrl_Pst/Ftn_SpdMtMethod/Nftn_ThetaOffset ==
  note: Input:
      | Description:
      | Output:
  i16PstNow : Inport  Description=■ 설명: 위치센서 카운트 신호 ( NOW )  OutMin=0  OutMax=4095
      settings: AttributesFormatString=%<Description>
  Add : Sum  Inputs=+-
  CB_E02PST_sPI2InvPPR : Constant  Value=E02PST.sPI2InvPPR
  CB_E02PST_sThetaOffset : Constant  Value=E02PST.sThetaOffset
  DataTypeConversion : DataTypeConversion  OutDataTypeStr=single  SaturateOnIntegerOverflow=off  RndMeth=Floor
  Product : Product
  sThetaIntegIn : Outport  Description=■ 설명: 위치 센서 카운트 ( Unit Delay ) + Offset 출력  OutMin=0  OutMax=6.2832
      settings: AttributesFormatString=%<Description>
  wires:
  CB_E02PST_sPI2InvPPR/1 -> Product/2
  Product/1 -> Add/1  "sTemp"
  CB_E02PST_sThetaOffset/1 -> Add/2
  Add/1 -> sThetaIntegIn/1  "sThetaIntegIn"
  i16PstNow/1 -> DataTypeConversion/1
  DataTypeConversion/1 -> Product/1  "sPstNow"

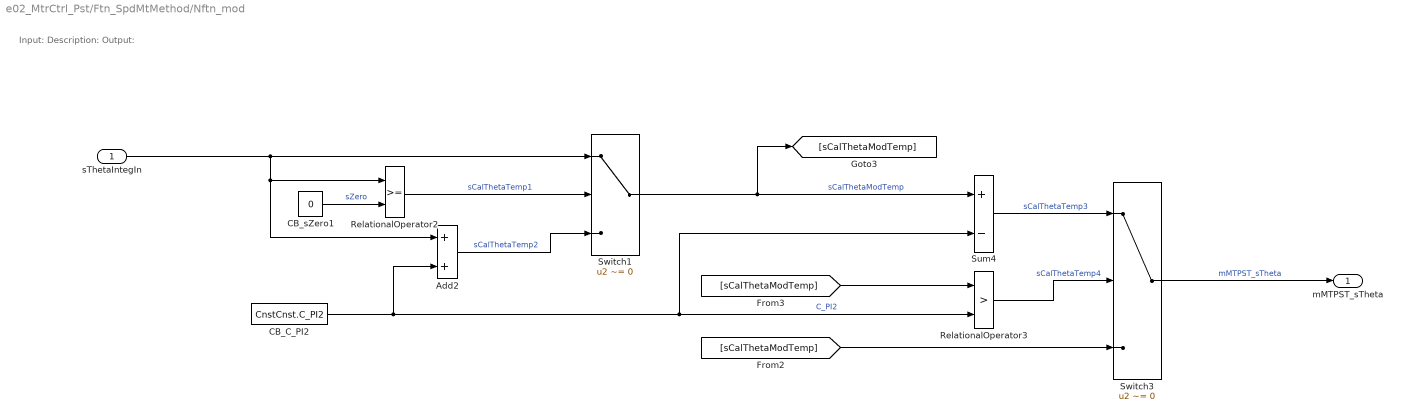
== system e02_MtrCtrl_Pst/Ftn_SpdMtMethod/Nftn_mod ==
  note: Input:
      | Description:
      | Output:
  sThetaIntegIn : Inport  Description=■ 설명: 위치 센서 카운트 ( Unit Delay ) + Offset 출력  OutMin=0  OutMax=6.2832
      settings: AttributesFormatString=%<Description>
  Add2 : Sum
  CB_C_PI2 : Constant  Value=CnstCnst.C_PI2
  CB_sZero1 : Constant  Value=0  OutDataTypeStr=single
  RelationalOperator2 : RelationalOperator  InputSameDT=off
  RelationalOperator3 : RelationalOperator  Operator=>  InputSameDT=off
  Sum4 : Sum  Inputs=+-
  Switch1 : Switch  Criteria=u2 ~= 0  SaturateOnIntegerOverflow=off  InputSameDT=off
  Switch3 : Switch  Criteria=u2 ~= 0  SaturateOnIntegerOverflow=off  InputSameDT=off
  mMTPST_sTheta : Outport  Description=■ 설명: 엔코더 위치  OutMin=0  OutMax=6.2832  VectorParamsAs1DForOutWhenUnconnected=off
      settings: AttributesFormatString=%<Description>
  wires:
  Switch3/1 -> mMTPST_sTheta/1  "mMTPST_sTheta"
  RelationalOperator3/1 -> Switch3/2  "sCalThetaTemp4"
  [sCalThetaModTemp] -> Switch3/3
  sThetaIntegIn/1 -> Add2/1, RelationalOperator2/1, Switch1/1
  CB_sZero1/1 -> RelationalOperator2/2  "sZero"
  Add2/1 -> Switch1/3  "sCalThetaTemp2"
  [sCalThetaModTemp] -> RelationalOperator3/1
  CB_C_PI2/1 -> Add2/2, RelationalOperator3/2, Sum4/2  "C_PI2"
  RelationalOperator2/1 -> Switch1/2  "sCalThetaTemp1"
  Sum4/1 -> Switch3/1  "sCalThetaTemp3"
  Switch1/1 -> Sum4/1, [sCalThetaModTemp]  "sCalThetaModTemp"

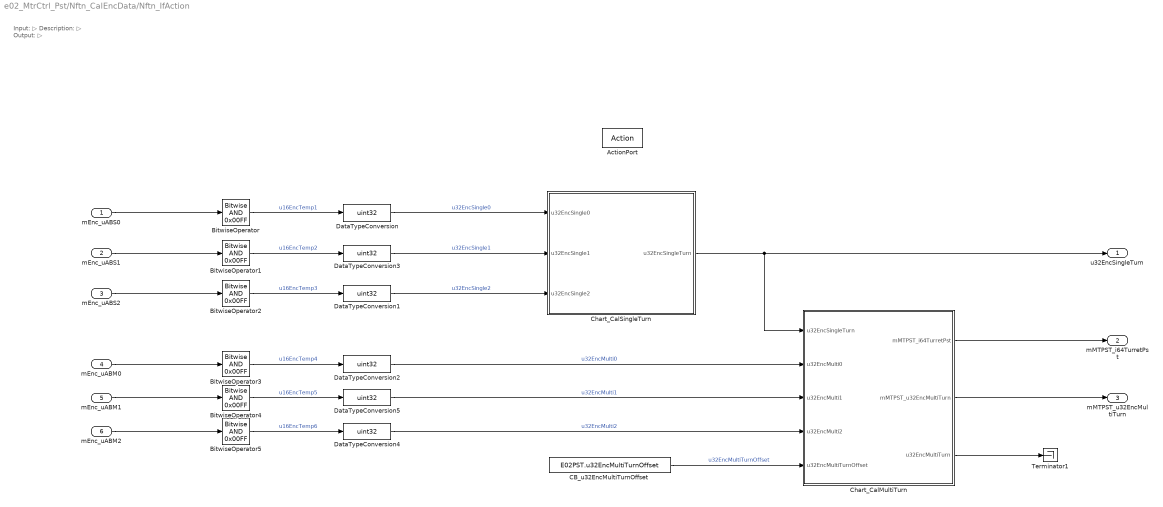
== system e02_MtrCtrl_Pst/Nftn_CalEncData/Nftn_IfAction ==
  note: Input:
      | ▷
      | Description:
      | ▷
      | Output:
      | ▷
  mEnc_uABS0 : Inport
  mEnc_uABS1 : Inport  Port=2
  mEnc_uABS2 : Inport  Port=3
  mEnc_uABM0 : Inport  Port=4
  mEnc_uABM1 : Inport  Port=5
  mEnc_uABM2 : Inport  Port=6
  ActionPort : ActionPort  ActionPortLabel=if(u1 == 35)
  BitwiseOperator{,1..5} (6 alike) : simulink/Logic and Bit Operations/Bitwise Operator  logicop=AND  UseBitMask=on  BitMask=0x00FF  BitMaskRealWorld=Stored Integer
  CB_u32EncMultiTurnOffset : Constant  Value=E02PST.u32EncMultiTurnOffset
  Chart_CalMultiTurn : Stateflow chart  TreatAsAtomicUnit=on
  Chart_CalSingleTurn : Stateflow chart  TreatAsAtomicUnit=on
  DataTypeConversion{,1..5} (6 alike) : DataTypeConversion  OutDataTypeStr=uint32  SaturateOnIntegerOverflow=off  RndMeth=Floor
  Terminator1 : Terminator
  u32EncSingleTurn : Outport
  mMTPST_i64TurretPst : Outport  Port=2
  mMTPST_u32EncMultiTurn : Outport  Port=3
  wires:
  BitwiseOperator/1 -> DataTypeConversion/1  "u16EncTemp1"
  BitwiseOperator5/1 -> DataTypeConversion4/1  "u16EncTemp6"
  mEnc_uABS2/1 -> BitwiseOperator2/1
  BitwiseOperator1/1 -> DataTypeConversion3/1  "u16EncTemp2"
  DataTypeConversion/1 -> Chart_CalSingleTurn/1(u32EncSingle0)  "u32EncSingle0"
  Chart_CalMultiTurn/3(u32EncMultiTurn) -> Terminator1/1
  DataTypeConversion2/1 -> Chart_CalMultiTurn/2(u32EncMulti0)  "u32EncMulti0"
  DataTypeConversion4/1 -> Chart_CalMultiTurn/4(u32EncMulti2)  "u32EncMulti2"
  DataTypeConversion1/1 -> Chart_CalSingleTurn/3(u32EncSingle2)  "u32EncSingle2"
  BitwiseOperator3/1 -> DataTypeConversion2/1  "u16EncTemp4"
  mEnc_uABM0/1 -> BitwiseOperator3/1
  BitwiseOperator4/1 -> DataTypeConversion5/1  "u16EncTemp5"
  BitwiseOperator2/1 -> DataTypeConversion1/1  "u16EncTemp3"
  DataTypeConversion5/1 -> Chart_CalMultiTurn/3(u32EncMulti1)  "u32EncMulti1"
  mEnc_uABM2/1 -> BitwiseOperator5/1
  DataTypeConversion3/1 -> Chart_CalSingleTurn/2(u32EncSingle1)  "u32EncSingle1"
  Chart_CalSingleTurn/1(u32EncSingleTurn) -> Chart_CalMultiTurn/1(u32EncSingleTurn), u32EncSingleTurn/1
  mEnc_uABS1/1 -> BitwiseOperator1/1
  mEnc_uABM1/1 -> BitwiseOperator4/1
  mEnc_uABS0/1 -> BitwiseOperator/1
  Chart_CalMultiTurn/2(mMTPST_u32EncMultiTurn) -> mMTPST_u32EncMultiTurn/1
  Chart_CalMultiTurn/1(mMTPST_i64TurretPst) -> mMTPST_i64TurretPst/1
  CB_u32EncMultiTurnOffset/1 -> Chart_CalMultiTurn/5(u32EncMultiTurnOffset)  "u32EncMultiTurnOffset"

== stateflow chart e02_MtrCtrl_Pst/Nftn_CalEncData/Nftn_IfAction/Chart_CalSingleTurn ==
  (default) -> (junction 1)
  (junction 1) -> (junction 3) : {
      | u32EncSingleTurn = u32EncSingle0 | (u32EncSingle1<<8) | (u32EncSingle2<<16);
      | }
  data: u32EncSingleTurn output uint32; u32EncSingle0 input; u32EncSingle1 input; u32EncSingle2 input

== stateflow chart e02_MtrCtrl_Pst/Ftn_RevAbc2dqe/Ftn_OverCurrDebounceFilter ==
  note: /* OC_Noise 발생시 이전 Idq 전류를 제어기에 적용 */
  (default) -> (junction 3)
  (junction 3) -> (junction 5) [order 1] : [mDIAG_uCntCrtOvr == uZero]
  (junction 3) -> (junction 6) [order 2] : /* no action */
  (junction 5) -> (junction 7) : {
      | mMTPST_sIde = sIdeTemp;
      | mMTPST_sIqe = sIqeTemp;
      | }
  (junction 7) -> (junction 6)
  (junction 6) -> (junction 12)
  data: mDIAG_uCntCrtOvr input; sIdeTemp input; uZero input; sIqeTemp input; mMTPST_sIde output single; mMTPST_sIqe output single

== stateflow chart e02_MtrCtrl_Pst/Ftn_SpdMtMethod/Ftn_CalMdata/Chart_CalMdata ==
  note: [(i16PstNow > i16AllowedCntMin) && (sSpdNowZ < sZero)]
  note: [(i16PstNow < -i16AllowedCntMin) && (sSpdNowZ > sZero)]
  (default) -> (junction 18)
  (junction 18) -> (junction 19) [order 1] : [i16PstNow > i16AllowedCntMin]
  (junction 18) -> (junction 20) [order 2]
  (junction 19) -> (junction 24) : {
      | i16Mdata = i16PstNow - i16EncElectMaxCnt;
      | }
  (junction 20) -> (junction 21) [order 1] : [i16PstNow < -i16AllowedCntMin]
  (junction 20) -> (junction 22) [order 2] : {
      | i16Mdata = i16PstNow;
      | }
  (junction 21) -> (junction 23) : {
      | i16Mdata = i16PstNow + i16EncElectMaxCnt;
      | }
  (junction 23) -> (junction 22)
  (junction 24) -> (junction 23)
  (junction 22) -> (junction 25)
  data: i16PstNow input; i16AllowedCntMin input; i16EncElectMaxCnt input; i16Mdata output int16

== stateflow chart e02_MtrCtrl_Pst/Nftn_CalEncData/Nftn_IfAction/Chart_CalMultiTurn ==
  note: if(ENC_multi_ORI > MULTI_OFFSET)
      | 				ENC_multi = ENC_multi_ORI - MULTI_OFFSET;
      | 			else
      | 				ENC_multi = ENC_multi_ORI + MULTI_OFFSET;
      |
      | 			Position = ((Uint64)ENC_single & 0x0001ffff) | ((Uint64)(ENC_multi & 0x0000ffff) << 17);
  (default) -> (junction 1)
  (junction 1) -> (junction 16) : {
      | mMTPST_u32EncMultiTurn = u32EncMulti0 | (u32EncMulti1<<8) | (u32EncMulti2<<16);
      | }
  (junction 16) -> (junction 17) [order 1] : [mMTPST_u32EncMultiTurn > u32EncMultiTurnOffset]
  (junction 16) -> (junction 18) [order 2] : {
      | u32EncMultiTurn = mMTPST_u32EncMultiTurn + u32EncMultiTurnOffset;
      | }
  (junction 17) -> (junction 19) : {
      | u32EncMultiTurn = mMTPST_u32EncMultiTurn - u32EncMultiTurnOffset;
      | }
  (junction 19) -> (junction 18)
  (junction 18) -> (junction 20) : {
      | mMTPST_i64TurretPst = int64(u32EncSingleTurn & 0x0001FFFF) | (int64(u32EncMultiTurn & 0x0000FFFF) << 17);
      | }
  data: mMTPST_i64TurretPst output int64; u32EncSingleTurn input; mMTPST_u32EncMultiTurn output uint32; u32EncMulti0 input; u32EncMulti1 input; u32EncMulti2 input; u32EncMultiTurn output uint32; u32EncMultiTurnOffset input
